simulink model "KUKA_LUNGU"  (R2016b)
settings: Solver=VariableStepAuto  StartTime=0  StopTime=inf  RelTol=1e-3
undefined symbols (not defined in the file or in its folder): KR16, KR16L1, KR16L2, KR16L3, KR16L4, KR16L5, KR16L6, KR16底座, KR16电主轴, KUKA, RootGround, RootPart
libraries: mblibv1 x42, simulink x7
settings Model: Creator=16591  LastModifiedBy=16591
settings SimMechanicsCC: VisOnUpdateDiagram=on  VisDuringSimulation=on

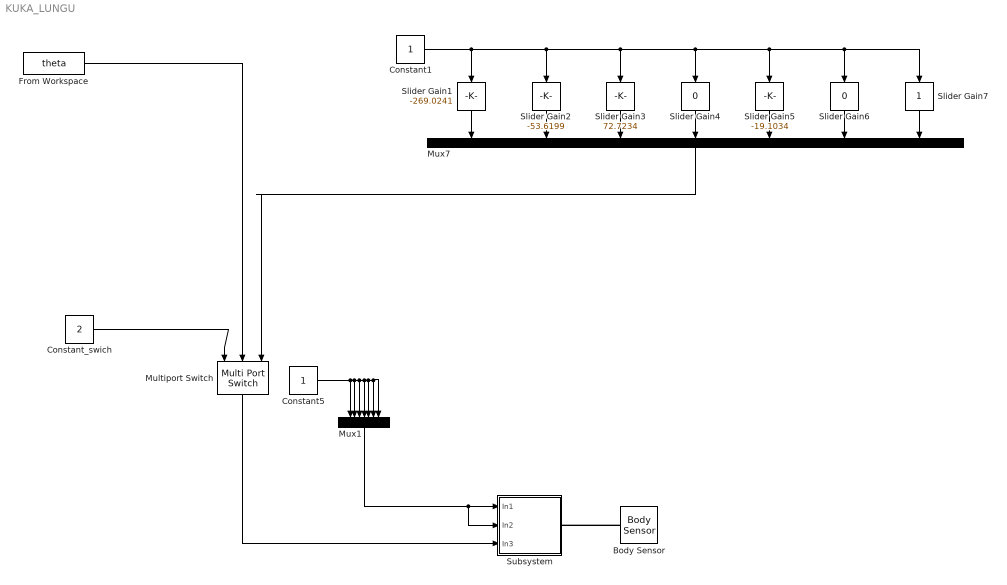
== system KUKA_LUNGU ==
  Body Sensor : mblibv1/Sensors &  Actuators/Body Sensor  UpdateFromCAD=off  PhysicalDomain=Mechanical  PortType=blob  Muxed=on  Pose=off  Angle=on  AngleUnits=deg  ArcVelocity=off  ArcVelocityUnits=deg/s  ArcAcceleration=off  ArcAccelerationUnits=deg/s^2  CoordPosition=on  CoordPositionUnits=m  Velocity=off  VelocityUnits=m/s  Acceleration=off  AccelerationUnits=m/s^2  Quaternion=on  QuaternionDT=off  QuaternionDDT=off  QuaternionUnits=off  OutputVector=[1]  ActiveIO=on  Width=3  DialogClass=MechanicalSensorBlock  ReferenceFrame=Absolute (World)
  Constant1 : Constant
  Constant5 : Constant
  Constant_swich : Constant  Value=2
  From Workspace : FromWorkspace  VariableName=theta  SampleTime=0.1
  Multiport Switch : MultiPortSwitch  Inputs=2
  Mux1 : Mux  Inputs=7
  Mux7 : Mux  Inputs=7
  Slider Gain1 : simulink/Math Operations/Slider Gain  low=-185  gain=-269.0241  high=185
  Slider Gain2 : simulink/Math Operations/Slider Gain  low=-155  gain=-53.6199  high=35
  Slider Gain3 : simulink/Math Operations/Slider Gain  low=-130  gain=72.7234  high=154
  Slider Gain4 : simulink/Math Operations/Slider Gain  low=-350  gain=0  high=350
  Slider Gain5 : simulink/Math Operations/Slider Gain  low=-130  gain=-19.1034  high=130
  Slider Gain6 : simulink/Math Operations/Slider Gain  low=-350  gain=0  high=350
  Slider Gain7 : simulink/Math Operations/Slider Gain  low=0  gain=1  high=2
  Subsystem : Subsystem
  wires:
  Multiport Switch/1 -> Subsystem/3(In3)
  Slider Gain1/1 -> Mux7/1
  Constant1/1 -> Slider Gain7/1, Slider Gain6/1, Slider Gain5/1, Slider Gain4/1, Slider Gain3/1, Slider Gain2/1, Slider Gain1/1
  Slider Gain2/1 -> Mux7/2
  Slider Gain3/1 -> Mux7/3
  Slider Gain4/1 -> Mux7/4
  Slider Gain5/1 -> Mux7/5
  Slider Gain6/1 -> Mux7/6
  Slider Gain7/1 -> Mux7/7
  Mux7/1 -> Multiport Switch/3
  Constant_swich/1 -> Multiport Switch/1
  Constant5/1 -> Mux1/1, Mux1/7, Mux1/6, Mux1/5, Mux1/4, Mux1/3, Mux1/2
  Mux1/1 -> Subsystem/2(In2), Subsystem/1(In1)
  From Workspace/1 -> Multiport Switch/2
  connections:
  Body Sensor/LConn1 -- Subsystem/RConn1

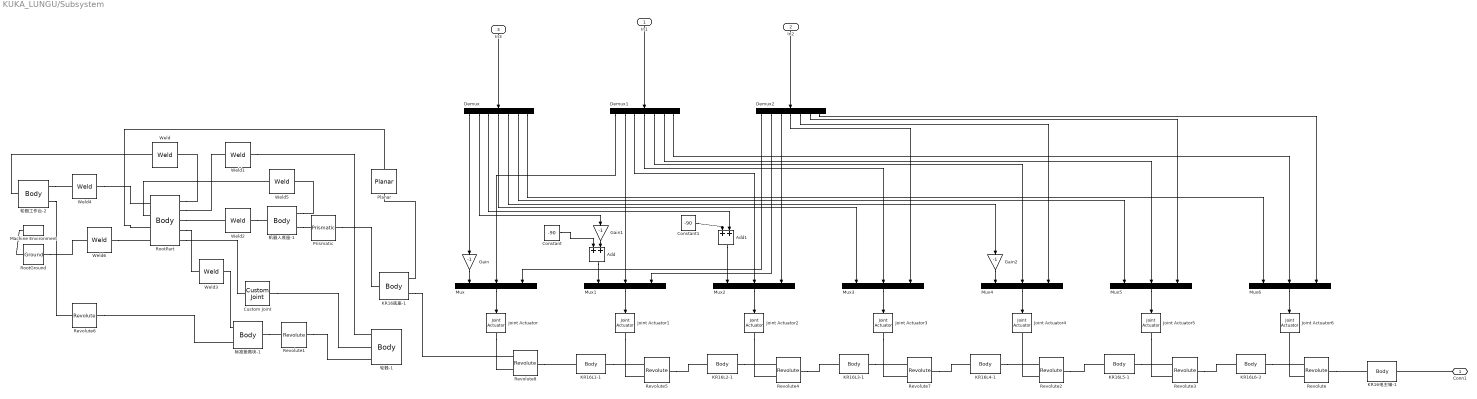
== system KUKA_LUNGU/Subsystem ==
  In1 : Inport
  In2 : Inport  Port=2
  In3 : Inport  Port=3
  Add : Sum
  Add1 : Sum
  Constant : Constant  Value=-90
  Constant1 : Constant  Value=-90
  Custom Joint : mblibv1/Joints/Custom Joint  LConnTagsString=__newl0  RConnTagsString=__newr0  UpdateFromCAD=on  PMImportedID=:-:KUKA-KR16-汽车轮毂/RootPart  NumSAPorts=0  CutJoint=off  MarkAsCut=off  Primitives=prismatic  PrimitiveProps=P1$WORLD$[1,0,0]$prismatic#P2$WORLD$[0,1,0]$prismatic#P3$WORLD$[0,0,1]$prismatic#R1$WORLD$[1,0,0]$revolute  DialogClass=JointBlock  R1Axis=[1,0,0]  R2Axis=[]  R3Axis=[]  P1Axis=[1,0,0]  P2Axis=[0,1,0]  P3Axis=[0,0,1]  SAxis=[]
  Demux : Demux  Outputs=7
  Demux1 : Demux  Outputs=7
  Demux2 : Demux  Outputs=7
  Gain : Gain  Gain=-1
  Gain1 : Gain  Gain=-1
  Gain2 : Gain  Gain=-1
  Joint Actuator{,1..6} (7 alike) : mblibv1/Sensors &  Actuators/Joint Actuator  UpdateFromCAD=off  PhysicalDomain=Mechanical  PortType=blob  ActuationStyle=Motion  AngleUnits=deg  ArcVelocityUnits=deg/s  ArcAccelerationUnits=deg/s^2  CoordPositionUnits=m  VelocityUnits=m/s  AccelerationUnits=m/s^2  ForceUnits=N  TorqueUnits=N*m  ActiveIO=on  Width=3  DialogClass=MechanicalActuatorBlock  Primitive=R1  ReferenceFrame=Absolute (World)
  KR16L1-1 : mblibv1/Bodies/Body  LConnTagsString=CS3  RConnTagsString=CS2  UpdateFromCAD=on  PMImportedID=KR16L1-1  DialogClass=MechanicalBodyBlock  Mass=25.8177  MassUnits=kg  InertiaUnits=kg*m^2  Inertia=[0.576803,-0.0576744,-0.301475;-0.0576744,0.906894,-0.0524576;-0.301475,-0.0524576,0.799958]  Shape=Cylinder  ShapeDims=[1 1]  ShapeUnits=m  ShapeUse=false  Density=1  DensityUnits=kg/m^3  DensityUse=false  GraphicsMode=GFXFILE  GraphicsFileName=KUKA-KR16-汽车轮毂 - KR16L1-1.STL  BodyColorSelMode=COLORPALETTE  BodyColor=[0.960784;0.419608;0.141176]  AttachedToCS=CS1  CG=Right$CG$[0.119444 1.06418 -0.0189084]$WORLD$WORLD$m$[1 0 0;0 0 1;0 -1 0]$3x3 Transform$rad$WORLD$false$KR16L1-1::CG(AUTOGEN)  WorkingFrames=Right$CS1$[0 0.5 0]$WORLD$WORLD$m$[1 0 0;0 0 1;0 -1 0]$3x3 Transform$rad$WORLD$false$KR16L1-1::CS1(AUTOGEN)#Right$CS2$[0.26 1.175 0.067]$WORLD$WORLD$m$[1 0 0;0 1 0;0 0 1]$3x3 Transform$rad$WORLD$true$KR16L1-1:-:KR16L2-1::KR16L1-1(AUTOGEN)#Left$CS3$[0 0.5474 0]$WORLD$WORLD$m$[1 0 0;0 1 0;0 0 1]$3x3 Transform$rad$WORLD$true$KR16L1-1:-:KR16底座-1::KR16L1-1(AUTOGEN)  CGPos=[0.119444 1.06418 -0.0189084]  CGRot=[1 0 0;0 0 1;0 -1 0]  CS0Pos=[]  CS0Rot=[]  CS1Pos=[0 0.5 0]  CS1Rot=[1 0 0;0 0 1;0 -1 0]  CS2Pos=[0.26 1.175 0.067]  CS2Rot=[1 0 0;0 1 0;0 0 1]  CS3Pos=[0 0.5474 0]  CS3Rot=[1 0 0;0 1 0;0 0 1]  CS4Pos=[]  CS4Rot=[]  CS5Pos=[]  CS5Rot=[]  CS6Pos=[]  CS6Rot=[]  CS7Pos=[]  CS7Rot=[]  CS8Pos=[]  CS8Rot=[]  CS9Pos=[]  CS9Rot=[]  CS10Pos=[]  CS10Rot=[]  CS11Pos=[]  CS11Rot=[]  CS12Pos=[]  CS12Rot=[]  CS13Pos=[]  CS13Rot=[]  CS14Pos=[]  CS14Rot=[]  CS15Pos=[]  CS15Rot=[]  CS16Pos=[]  CS16Rot=[]  CS17Pos=[]  CS17Rot=[]  CS18Pos=[]  CS18Rot=[]  CS19Pos=[]  CS19Rot=[]  CS20Pos=[]  CS20Rot=[]
  KR16L2-1 : mblibv1/Bodies/Body  LConnTagsString=CS3  RConnTagsString=CS2  UpdateFromCAD=on  PMImportedID=KR16L2-1  DialogClass=MechanicalBodyBlock  Mass=13.4955  MassUnits=kg  InertiaUnits=kg*m^2  Inertia=[0.593067,-0.000241705,-0.000338834;-0.000241705,0.591348,0.0261399;-0.000338834,0.0261399,0.0591147]  Shape=Cylinder  ShapeDims=[1 1]  ShapeUnits=m  ShapeUse=false  Density=1  DensityUnits=kg/m^3  DensityUse=false  GraphicsMode=GFXFILE  GraphicsFileName=KUKA-KR16-汽车轮毂 - KR16L2-1.STL  BodyColorSelMode=COLORPALETTE  BodyColor=[0.960784;0.419608;0.141176]  AttachedToCS=CS1  CG=Right$CG$[0.260237 1.49663 0.180665]$WORLD$WORLD$m$[1 0 -5.63789e-11;5.63789e-11 0 1;0 -1 0]$3x3 Transform$rad$WORLD$false$KR16L2-1::CG(AUTOGEN)  WorkingFrames=Right$CS1$[3.8056e-11 0.5 0]$WORLD$WORLD$m$[1 0 -5.63789e-11;5.63789e-11 0 1;0 -1 0]$3x3 Transform$rad$WORLD$false$KR16L2-1::CS1(AUTOGEN)#Right$CS2$[0.26 1.855 0.107]$WORLD$WORLD$m$[1 0 0;0 1 0;0 0 1]$3x3 Transform$rad$WORLD$true$KR16L2-1:-:KR16L3-1::KR16L2-1(AUTOGEN)#Left$CS3$[0.26 1.175 0.067]$WORLD$WORLD$m$[1 0 0;0 1 0;0 0 1]$3x3 Transform$rad$WORLD$true$KR16L1-1:-:KR16L2-1::KR16L2-1(AUTOGEN)  CGPos=[0.260237 1.49663 0.180665]  CGRot=[1 0 -5.63789e-11;5.63789e-11 0 1;0 -1 0]  CS0Pos=[]  CS0Rot=[]  CS1Pos=[3.8056e-11 0.5 0]  CS1Rot=[1 0 -5.63789e-11;5.63789e-11 0 1;0 -1 0]  CS2Pos=[0.26 1.855 0.107]  CS2Rot=[1 0 0;0 1 0;0 0 1]  CS3Pos=[0.26 1.175 0.067]  CS3Rot=[1 0 0;0 1 0;0 0 1]  CS4Pos=[]  CS4Rot=[]  CS5Pos=[]  CS5Rot=[]  CS6Pos=[]  CS6Rot=[]  CS7Pos=[]  CS7Rot=[]  CS8Pos=[]  CS8Rot=[]  CS9Pos=[]  CS9Rot=[]  CS10Pos=[]  CS10Rot=[]  CS11Pos=[]  CS11Rot=[]  CS12Pos=[]  CS12Rot=[]  CS13Pos=[]  CS13Rot=[]  CS14Pos=[]  CS14Rot=[]  CS15Pos=[]  CS15Rot=[]  CS16Pos=[]  CS16Rot=[]  CS17Pos=[]  CS17Rot=[]  CS18Pos=[]  CS18Rot=[]  CS19Pos=[]  CS19Rot=[]  CS20Pos=[]  CS20Rot=[]
  KR16L3-1 : mblibv1/Bodies/Body  LConnTagsString=CS2  RConnTagsString=CS3  UpdateFromCAD=on  PMImportedID=KR16L3-1  DialogClass=MechanicalBodyBlock  Mass=16.2699  MassUnits=kg  InertiaUnits=kg*m^2  Inertia=[0.125403,0.00230248,0.000189371;0.00230248,0.543915,-0.00277001;0.000189371,-0.00277001,0.558145]  Shape=Cylinder  ShapeDims=[1 1]  ShapeUnits=m  ShapeUse=false  Density=1  DensityUnits=kg/m^3  DensityUse=false  GraphicsMode=GFXFILE  GraphicsFileName=KUKA-KR16-汽车轮毂 - KR16L3-1.STL  BodyColorSelMode=COLORPALETTE  BodyColor=[0.960784;0.419608;0.141176]  AttachedToCS=CS1  CG=Right$CG$[0.262138 1.83547 -0.00994259]$WORLD$WORLD$m$[1 0 -6.72099e-11;6.72099e-11 0 1;0 -1 0]$3x3 Transform$rad$WORLD$false$KR16L3-1::CG(AUTOGEN)  WorkingFrames=Right$CS1$[5.2732e-11 0.5 0]$WORLD$WORLD$m$[1 0 -6.72099e-11;6.72099e-11 0 1;0 -1 0]$3x3 Transform$rad$WORLD$false$KR16L3-1::CS1(AUTOGEN)#Left$CS2$[0.26 1.855 0.107]$WORLD$WORLD$m$[1 0 0;0 1 0;0 0 1]$3x3 Transform$rad$WORLD$true$KR16L2-1:-:KR16L3-1::KR16L3-1(AUTOGEN)#Right$CS3$[0.111 1.82 0]$WORLD$WORLD$m$[1 0 0;0 1 0;0 0 1]$3x3 Transform$rad$WORLD$true$KR16L3-1:-:KR16L4-1::KR16L3-1(AUTOGEN)  CGPos=[0.262138 1.83547 -0.00994259]  CGRot=[1 0 -6.72099e-11;6.72099e-11 0 1;0 -1 0]  CS0Pos=[]  CS0Rot=[]  CS1Pos=[5.2732e-11 0.5 0]  CS1Rot=[1 0 -6.72099e-11;6.72099e-11 0 1;0 -1 0]  CS2Pos=[0.26 1.855 0.107]  CS2Rot=[1 0 0;0 1 0;0 0 1]  CS3Pos=[0.111 1.82 0]  CS3Rot=[1 0 0;0 1 0;0 0 1]  CS4Pos=[]  CS4Rot=[]  CS5Pos=[]  CS5Rot=[]  CS6Pos=[]  CS6Rot=[]  CS7Pos=[]  CS7Rot=[]  CS8Pos=[]  CS8Rot=[]  CS9Pos=[]  CS9Rot=[]  CS10Pos=[]  CS10Rot=[]  CS11Pos=[]  CS11Rot=[]  CS12Pos=[]  CS12Rot=[]  CS13Pos=[]  CS13Rot=[]  CS14Pos=[]  CS14Rot=[]  CS15Pos=[]  CS15Rot=[]  CS16Pos=[]  CS16Rot=[]  CS17Pos=[]  CS17Rot=[]  CS18Pos=[]  CS18Rot=[]  CS19Pos=[]  CS19Rot=[]  CS20Pos=[]  CS20Rot=[]
  KR16L4-1 : mblibv1/Bodies/Body  LConnTagsString=CS3  RConnTagsString=CS2  UpdateFromCAD=on  PMImportedID=KR16L4-1  DialogClass=MechanicalBodyBlock  Mass=3.83148  MassUnits=kg  InertiaUnits=kg*m^2  Inertia=[0.00881654,-0.00289828,3.03725e-06;-0.00289828,0.0376269,-2.2375e-05;3.03725e-06,-2.2375e-05,0.0382811]  Shape=Cylinder  ShapeDims=[1 1]  ShapeUnits=m  ShapeUse=false  Density=1  DensityUnits=kg/m^3  DensityUse=false  GraphicsMode=GFXFILE  GraphicsFileName=KUKA-KR16-汽车轮毂 - KR16L4-1.STL  BodyColorSelMode=COLORPALETTE  BodyColor=[0.960784;0.419608;0.141176]  AttachedToCS=CS1  CG=Right$CG$[0.794534 1.81999 -0.00555632]$WORLD$WORLD$m$[1 0 -6.72102e-11;6.72101e-11 -5.18527e-12 1;0 -1 -5.18528e-12]$3x3 Transform$rad$WORLD$false$KR16L4-1::CG(AUTOGEN)  WorkingFrames=Right$CS1$[5.27326e-11 0.5 7.41978e-12]$WORLD$WORLD$m$[1 0 -6.72102e-11;6.72101e-11 -5.18527e-12 1;0 -1 -5.18528e-12]$3x3 Transform$rad$WORLD$false$KR16L4-1::CS1(AUTOGEN)#Right$CS2$[0.93 1.82 0.0335]$WORLD$WORLD$m$[1 0 0;0 1 0;0 0 1]$3x3 Transform$rad$WORLD$true$KR16L4-1:-:KR16L5-1::KR16L4-1(AUTOGEN)#Left$CS3$[0.111 1.82 0]$WORLD$WORLD$m$[1 0 0;0 1 0;0 0 1]$3x3 Transform$rad$WORLD$true$KR16L3-1:-:KR16L4-1::KR16L4-1(AUTOGEN)  CGPos=[0.794534 1.81999 -0.00555632]  CGRot=[1 0 -6.72102e-11;6.72101e-11 -5.18527e-12 1;0 -1 -5.18528e-12]  CS0Pos=[]  CS0Rot=[]  CS1Pos=[5.27326e-11 0.5 7.41978e-12]  CS1Rot=[1 0 -6.72102e-11;6.72101e-11 -5.18527e-12 1;0 -1 -5.18528e-12]  CS2Pos=[0.93 1.82 0.0335]  CS2Rot=[1 0 0;0 1 0;0 0 1]  CS3Pos=[0.111 1.82 0]  CS3Rot=[1 0 0;0 1 0;0 0 1]  CS4Pos=[]  CS4Rot=[]  CS5Pos=[]  CS5Rot=[]  CS6Pos=[]  CS6Rot=[]  CS7Pos=[]  CS7Rot=[]  CS8Pos=[]  CS8Rot=[]  CS9Pos=[]  CS9Rot=[]  CS10Pos=[]  CS10Rot=[]  CS11Pos=[]  CS11Rot=[]  CS12Pos=[]  CS12Rot=[]  CS13Pos=[]  CS13Rot=[]  CS14Pos=[]  CS14Rot=[]  CS15Pos=[]  CS15Rot=[]  CS16Pos=[]  CS16Rot=[]  CS17Pos=[]  CS17Rot=[]  CS18Pos=[]  CS18Rot=[]  CS19Pos=[]  CS19Rot=[]  CS20Pos=[]  CS20Rot=[]
  KR16L5-1 : mblibv1/Bodies/Body  LConnTagsString=CS2  RConnTagsString=CS3  UpdateFromCAD=on  PMImportedID=KR16L5-1  DialogClass=MechanicalBodyBlock  Mass=1.85731  MassUnits=kg  InertiaUnits=kg*m^2  Inertia=[0.008719,0.000329435,2.41862e-07;0.000329435,0.00689293,-1.21594e-06;2.41862e-07,-1.21594e-06,0.012927]  Shape=Cylinder  ShapeDims=[1 1]  ShapeUnits=m  ShapeUse=false  Density=1  DensityUnits=kg/m^3  DensityUse=false  GraphicsMode=GFXFILE  GraphicsFileName=KUKA-KR16-汽车轮毂 - KR16L5-1.STL  BodyColorSelMode=COLORPALETTE  BodyColor=[0.960784;0.419608;0.141176]  AttachedToCS=CS1  CG=Right$CG$[0.930049 1.7697 0.0071318]$WORLD$WORLD$m$[4.40623e-11 1.89374e-10 1;-1 -5.18503e-12 4.40623e-11;5.18503e-12 -1 1.89374e-10]$3x3 Transform$rad$WORLD$false$KR16L5-1::CG(AUTOGEN)  WorkingFrames=Right$CS1$[-0.39 2.75 -2.54769e-10]$WORLD$WORLD$m$[4.40623e-11 1.89374e-10 1;-1 -5.18503e-12 4.40623e-11;5.18503e-12 -1 1.89374e-10]$3x3 Transform$rad$WORLD$false$KR16L5-1::CS1(AUTOGEN)#Left$CS2$[0.93 1.82 0.0335]$WORLD$WORLD$m$[1 0 0;0 1 0;0 0 1]$3x3 Transform$rad$WORLD$true$KR16L4-1:-:KR16L5-1::KR16L5-1(AUTOGEN)#Right$CS3$[0.93 1.662 7.32896e-11]$WORLD$WORLD$m$[1 0 0;0 1 0;0 0 1]$3x3 Transform$rad$WORLD$true$KR16L5-1:-:KR16L6-3::KR16L5-1(AUTOGEN)  CGPos=[0.930049 1.7697 0.0071318]  CGRot=[4.40623e-11 1.89374e-10 1;-1 -5.18503e-12 4.40623e-11;5.18503e-12 -1 1.89374e-10]  CS0Pos=[]  CS0Rot=[]  CS1Pos=[-0.39 2.75 -2.54769e-10]  CS1Rot=[4.40623e-11 1.89374e-10 1;-1 -5.18503e-12 4.40623e-11;5.18503e-12 -1 1.89374e-10]  CS2Pos=[0.93 1.82 0.0335]  CS2Rot=[1 0 0;0 1 0;0 0 1]  CS3Pos=[0.93 1.662 7.32896e-11]  CS3Rot=[1 0 0;0 1 0;0 0 1]  CS4Pos=[]  CS4Rot=[]  CS5Pos=[]  CS5Rot=[]  CS6Pos=[]  CS6Rot=[]  CS7Pos=[]  CS7Rot=[]  CS8Pos=[]  CS8Rot=[]  CS9Pos=[]  CS9Rot=[]  CS10Pos=[]  CS10Rot=[]  CS11Pos=[]  CS11Rot=[]  CS12Pos=[]  CS12Rot=[]  CS13Pos=[]  CS13Rot=[]  CS14Pos=[]  CS14Rot=[]  CS15Pos=[]  CS15Rot=[]  CS16Pos=[]  CS16Rot=[]  CS17Pos=[]  CS17Rot=[]  CS18Pos=[]  CS18Rot=[]  CS19Pos=[]  CS19Rot=[]  CS20Pos=[]  CS20Rot=[]
  KR16L6-3 : mblibv1/Bodies/Body  LConnTagsString=CS3  RConnTagsString=CS2  UpdateFromCAD=on  PMImportedID=KR16L6-3  DialogClass=MechanicalBodyBlock  Mass=1.24036  MassUnits=kg  InertiaUnits=kg*m^2  Inertia=[0.00519585,0,0;0,0.00167069,0;0,0,0.00515745]  Shape=Cylinder  ShapeDims=[1 1]  ShapeUnits=m  ShapeUse=false  Density=1  DensityUnits=kg/m^3  DensityUse=false  GraphicsMode=GFXFILE  GraphicsFileName=KUKA-KR16-汽车轮毂 - KR16L6-3.STL  BodyColorSelMode=COLORPALETTE  BodyColor=[0.529412;0.54902;0.54902]  AttachedToCS=CS1  CG=Right$CG$[0.93 1.57551 7.3738e-11]$WORLD$WORLD$m$[0 -4.40624e-11 -1;5.1849e-12 1 -4.40623e-11;1 -5.18491e-12 0]$3x3 Transform$rad$WORLD$false$KR16L6-3::CG(AUTOGEN)  WorkingFrames=Right$CS1$[0.93 1.462 7.43266e-11]$WORLD$WORLD$m$[0 -4.40624e-11 -1;5.1849e-12 1 -4.40623e-11;1 -5.18491e-12 0]$3x3 Transform$rad$WORLD$false$KR16L6-3::CS1(AUTOGEN)#Right$CS2$[0.93 1.618 7.35177e-11]$WORLD$WORLD$m$[1 0 0;0 1 0;0 0 1]$3x3 Transform$rad$WORLD$true$KR16L6-3:-:KR16电主轴-1::KR16L6-3(AUTOGEN)#Left$CS3$[0.93 1.662 7.32896e-11]$WORLD$WORLD$m$[1 0 0;0 1 0;0 0 1]$3x3 Transform$rad$WORLD$true$KR16L5-1:-:KR16L6-3::KR16L6-3(AUTOGEN)  CGPos=[0.93 1.57551 7.3738e-11]  CGRot=[0 -4.40624e-11 -1;5.1849e-12 1 -4.40623e-11;1 -5.18491e-12 0]  CS0Pos=[]  CS0Rot=[]  CS1Pos=[0.93 1.462 7.43266e-11]  CS1Rot=[0 -4.40624e-11 -1;5.1849e-12 1 -4.40623e-11;1 -5.18491e-12 0]  CS2Pos=[0.93 1.618 7.35177e-11]  CS2Rot=[1 0 0;0 1 0;0 0 1]  CS3Pos=[0.93 1.662 7.32896e-11]  CS3Rot=[1 0 0;0 1 0;0 0 1]  CS4Pos=[]  CS4Rot=[]  CS5Pos=[]  CS5Rot=[]  CS6Pos=[]  CS6Rot=[]  CS7Pos=[]  CS7Rot=[]  CS8Pos=[]  CS8Rot=[]  CS9Pos=[]  CS9Rot=[]  CS10Pos=[]  CS10Rot=[]  CS11Pos=[]  CS11Rot=[]  CS12Pos=[]  CS12Rot=[]  CS13Pos=[]  CS13Rot=[]  CS14Pos=[]  CS14Rot=[]  CS15Pos=[]  CS15Rot=[]  CS16Pos=[]  CS16Rot=[]  CS17Pos=[]  CS17Rot=[]  CS18Pos=[]  CS18Rot=[]  CS19Pos=[]  CS19Rot=[]  CS20Pos=[]  CS20Rot=[]
  KR16底座-1 : mblibv1/Bodies/Body  LConnTagsString=CS3  RConnTagsString=CS2|CS4  UpdateFromCAD=on  PMImportedID=KR16底座-1  DialogClass=MechanicalBodyBlock  Mass=70.1358  MassUnits=kg  InertiaUnits=kg*m^2  Inertia=[1.74612,0.032286,-0.0123849;0.032286,2.12719,-0.000120145;-0.0123849,-0.000120145,2.2593]  Shape=Cylinder  ShapeDims=[1 1]  ShapeUnits=m  ShapeUse=false  Density=1  DensityUnits=kg/m^3  DensityUse=false  GraphicsMode=GFXFILE  GraphicsFileName=KUKA-KR16-汽车轮毂 - KR16底座-1.STL  BodyColorSelMode=COLORPALETTE  BodyColor=[0.14902;0.14902;0.14902]  AttachedToCS=CS1  CG=Right$CG$[-0.0392869 0.697192 -0.00150494]$WORLD$WORLD$m$[1 0 0;0 0 1;0 -1 0]$3x3 Transform$rad$WORLD$false$KR16底座-1::CG(AUTOGEN)  WorkingFrames=Right$CS1$[0 0.5 0]$WORLD$WORLD$m$[1 0 0;0 0 1;0 -1 0]$3x3 Transform$rad$WORLD$false$KR16底座-1::CS1(AUTOGEN)#Right$CS2$[0 0.5 0]$WORLD$WORLD$m$[1 0 0;0 1 0;0 0 1]$3x3 Transform$rad$WORLD$true$:-:KUKA-KR16-汽车轮毂/RootPart::KR16底座-1(AUTOGEN)#Left$CS3$[0 0.5 0]$WORLD$WORLD$m$[1 0 0;0 1 0;0 0 1]$3x3 Transform$rad$WORLD$true$KR16底座-1:-:机器人底座-1::KR16底座-1(AUTOGEN)#Right$CS4$[0 0.5474 0]$WORLD$WORLD$m$[1 0 0;0 1 0;0 0 1]$3x3 Transform$rad$WORLD$true$KR16L1-1:-:KR16底座-1::KR16底座-1(AUTOGEN)  CGPos=[-0.0392869 0.697192 -0.00150494]  CGRot=[1 0 0;0 0 1;0 -1 0]  CS0Pos=[]  CS0Rot=[]  CS1Pos=[0 0.5 0]  CS1Rot=[1 0 0;0 0 1;0 -1 0]  CS2Pos=[0 0.5 0]  CS2Rot=[1 0 0;0 1 0;0 0 1]  CS3Pos=[0 0.5 0]  CS3Rot=[1 0 0;0 1 0;0 0 1]  CS4Pos=[0 0.5474 0]  CS4Rot=[1 0 0;0 1 0;0 0 1]  CS5Pos=[]  CS5Rot=[]  CS6Pos=[]  CS6Rot=[]  CS7Pos=[]  CS7Rot=[]  CS8Pos=[]  CS8Rot=[]  CS9Pos=[]  CS9Rot=[]  CS10Pos=[]  CS10Rot=[]  CS11Pos=[]  CS11Rot=[]  CS12Pos=[]  CS12Rot=[]  CS13Pos=[]  CS13Rot=[]  CS14Pos=[]  CS14Rot=[]  CS15Pos=[]  CS15Rot=[]  CS16Pos=[]  CS16Rot=[]  CS17Pos=[]  CS17Rot=[]  CS18Pos=[]  CS18Rot=[]  CS19Pos=[]  CS19Rot=[]  CS20Pos=[]  CS20Rot=[]
  KR16电主轴-1 : mblibv1/Bodies/Body  LConnTagsString=CS2  RConnTagsString=CS3  UpdateFromCAD=on  PMImportedID=KR16电主轴-1  DialogClass=MechanicalBodyBlock  Mass=0.0101259  MassUnits=kg  InertiaUnits=kg*m^2  Inertia=[2.07229e-06,0,0;0,4.76675e-07,0;0,0,2.07229e-06]  Shape=Cylinder  ShapeDims=[1 1]  ShapeUnits=m  ShapeUse=false  Density=1  DensityUnits=kg/m^3  DensityUse=false  GraphicsMode=GFXFILE  GraphicsFileName=KUKA-KR16-汽车轮毂 - KR16电主轴-1.STL  BodyColorSelMode=COLORPALETTE  BodyColor=[1;0;0]  AttachedToCS=CS1  CG=Right$CG$[0.93 1.44419 7.44189e-11]$WORLD$WORLD$m$[-0.760403 -4.40624e-11 -0.649452;-3.01378e-11 1 -3.2559e-11;0.649452 -5.18491e-12 -0.760403]$3x3 Transform$rad$WORLD$false$KR16电主轴-1::CG(AUTOGEN)  WorkingFrames=Right$CS3$[0.93 1.44419 7.44189e-11]$WORLD$WORLD$m$[-0.760403 -4.40624e-11 -0.649452;-3.01378e-11 1 -3.2559e-11;0.649452 -5.18491e-12 -0.760403]$3x3 Transform$rad$WORLD$true$none#Right$CS1$[0.93 1.402 7.46377e-11]$WORLD$WORLD$m$[-0.760403 -4.40624e-11 -0.649452;-3.01378e-11 1 -3.2559e-11;0.649452 -5.18491e-12 -0.760403]$3x3 Transform$rad$WORLD$false$KR16电主轴-1::CS1(AUTOGEN)#Left$CS2$[0.93 1.618 7.35177e-11]$WORLD$WORLD$m$[1 0 0;0 1 0;0 0 1]$3x3 Transform$rad$WORLD$true$KR16L6-3:-:KR16电主轴-1::KR16电主轴-1(AUTOGEN)  CGPos=[0.93 1.44419 7.44189e-11]  CGRot=[-0.760403 -4.40624e-11 -0.649452;-3.01378e-11 1 -3.2559e-11;0.649452 -5.18491e-12 -0.760403]  CS0Pos=[]  CS0Rot=[]  CS1Pos=[0.93 1.402 7.46377e-11]  CS1Rot=[-0.760403 -4.40624e-11 -0.649452;-3.01378e-11 1 -3.2559e-11;0.649452 -5.18491e-12 -0.760403]  CS2Pos=[0.93 1.618 7.35177e-11]  CS2Rot=[1 0 0;0 1 0;0 0 1]  CS3Pos=[0.93 1.44419 7.44189e-11]  CS3Rot=[-0.760403 -4.40624e-11 -0.649452;-3.01378e-11 1 -3.2559e-11;0.649452 -5.18491e-12 -0.760403]  CS4Pos=[]  CS4Rot=[]  CS5Pos=[]  CS5Rot=[]  CS6Pos=[]  CS6Rot=[]  CS7Pos=[]  CS7Rot=[]  CS8Pos=[]  CS8Rot=[]  CS9Pos=[]  CS9Rot=[]  CS10Pos=[]  CS10Rot=[]  CS11Pos=[]  CS11Rot=[]  CS12Pos=[]  CS12Rot=[]  CS13Pos=[]  CS13Rot=[]  CS14Pos=[]  CS14Rot=[]  CS15Pos=[]  CS15Rot=[]  CS16Pos=[]  CS16Rot=[]  CS17Pos=[]  CS17Rot=[]  CS18Pos=[]  CS18Rot=[]  CS19Pos=[]  CS19Rot=[]  CS20Pos=[]  CS20Rot=[]
  Machine Environment : mblibv1/Bodies/Machine Environment  PortType=env  PhysicalDomain=Mechanical  DialogTemplateClass=MECH.MachineEnvironment  SyncWhenCopied=off  Gravity=[0 -9.81 0]  GravityUnits=m/s^2  GravityAsSignal=off  Dimensionality=Auto-detect  AnalysisType=Forward dynamics  LinearAssemblyTolerance=1e-3  LinearAssemblyToleranceUnits=m  AngularAssemblyTolerance=1e-3  AngularAssemblyToleranceUnits=rad  ConstraintSolverType=Stabilizing  ConstraintRelTolerance=1e-4  ConstraintAbsTolerance=1e-4  UseRobustSingularityHandling=off  RedundancyAnalysisToleranceType=Automatically select tolerance  RedundancyAnalysisTolerance=1e-14  StatePerturbationType=Fixed  PerturbationSize=1e-5  VisualizeMachine=on  BodyVisualizationType=Use model default body geometries  BodyColorSelMode=Use model default  DefaultBodyColor=[1 0 0]
  Mux{,1..6} (7 alike) : Mux  Inputs=3
  Planar : mblibv1/Joints/Planar  LConnTagsString=__newl0  RConnTagsString=__newr0  UpdateFromCAD=on  PMImportedID=:-:KUKA-KR16-汽车轮毂/RootPart  NumSAPorts=0  CutJoint=off  MarkAsCut=off  Primitives=prismatic_prismatic  PrimitiveProps=P1$WORLD$[-1,0,0]$prismatic#P2$WORLD$[0,-1,0]$prismatic#R1$WORLD$[0,0,-1]$revolute  DialogClass=JointBlock  P1Axis=[-1,0,0]  P2Axis=[0,-1,0]  R1Axis=[0,0,-1]
  Prismatic : mblibv1/Joints/Prismatic  LConnTagsString=__newl0  RConnTagsString=__newr0  UpdateFromCAD=on  PMImportedID=KR16底座-1:-:机器人底座-1  NumSAPorts=0  CutJoint=off  MarkAsCut=off  Primitives=prismatic  PrimitiveProps=P1$WORLD$[0,0,1]$prismatic  DialogClass=JointBlock  P1Axis=[0,0,1]
  Revolute : mblibv1/Joints/Revolute  LConnTagsString=__newl0|SA1  RConnTagsString=__newr0  UpdateFromCAD=on  PMImportedID=KR16L6-3:-:KR16电主轴-1  NumSAPorts=1  CutJoint=off  MarkAsCut=off  Primitives=prismatic  PrimitiveProps=R1$World$[4.40624e-11,-1,5.18492e-12]$revolute  DialogClass=JointBlock  R1Axis=[4.40624e-11,-1,5.18492e-12]
  Revolute1 : mblibv1/Joints/Revolute  LConnTagsString=__newl0  RConnTagsString=__newr0  UpdateFromCAD=on  PMImportedID=标准垫高块-1:-:轮毂-1  NumSAPorts=0  CutJoint=off  MarkAsCut=off  Primitives=prismatic  PrimitiveProps=R1$WORLD$[0,1,0]$revolute  DialogClass=JointBlock  R1Axis=[0,1,0]
  Revolute2 : mblibv1/Joints/Revolute  LConnTagsString=__newl0|SA1  RConnTagsString=__newr0  UpdateFromCAD=on  PMImportedID=KR16L4-1:-:KR16L5-1  NumSAPorts=1  CutJoint=off  MarkAsCut=off  Primitives=prismatic  PrimitiveProps=R1$World$[-1.89374e-10,5.18525e-12,1]$revolute  DialogClass=JointBlock  R1Axis=[-1.89374e-10,5.18525e-12,1]
  Revolute3 : mblibv1/Joints/Revolute  LConnTagsString=__newl0|SA1  RConnTagsString=__newr0  UpdateFromCAD=on  PMImportedID=KR16L5-1:-:KR16L6-3  NumSAPorts=1  CutJoint=off  MarkAsCut=off  Primitives=prismatic  PrimitiveProps=R1$World$[-4.40623e-11,1,-5.18503e-12]$revolute  DialogClass=JointBlock  R1Axis=[-4.40623e-11,1,-5.18503e-12]
  Revolute4 : mblibv1/Joints/Revolute  LConnTagsString=__newl0|SA1  RConnTagsString=__newr0  UpdateFromCAD=on  PMImportedID=KR16L2-1:-:KR16L3-1  NumSAPorts=1  CutJoint=off  MarkAsCut=off  Primitives=prismatic  PrimitiveProps=R1$World$[0,0,-1]$revolute  DialogClass=JointBlock  R1Axis=[0,0,-1]
  Revolute5 : mblibv1/Joints/Revolute  LConnTagsString=__newl0|SA1  RConnTagsString=__newr0  UpdateFromCAD=on  PMImportedID=KR16L1-1:-:KR16L2-1  NumSAPorts=1  CutJoint=off  MarkAsCut=off  Primitives=prismatic  PrimitiveProps=R1$World$[0,0,1]$revolute  DialogClass=JointBlock  R1Axis=[0,0,1]
  Revolute6 : mblibv1/Joints/Revolute  LConnTagsString=__newl0  RConnTagsString=__newr0  UpdateFromCAD=on  PMImportedID=标准垫高块-1:-:轮毂工作台-2  NumSAPorts=0  CutJoint=off  MarkAsCut=off  Primitives=prismatic  PrimitiveProps=R1$WORLD$[0,1,0]$revolute  DialogClass=JointBlock  R1Axis=[0,1,0]
  Revolute7 : mblibv1/Joints/Revolute  LConnTagsString=__newl0|SA1  RConnTagsString=__newr0  UpdateFromCAD=on  PMImportedID=KR16L3-1:-:KR16L4-1  NumSAPorts=1  CutJoint=off  MarkAsCut=off  Primitives=prismatic  PrimitiveProps=R1$World$[1,6.72099e-11,0]$revolute  DialogClass=JointBlock  R1Axis=[1,6.72099e-11,0]
  Revolute8 : mblibv1/Joints/Revolute  LConnTagsString=__newl0|SA1  RConnTagsString=__newr0  UpdateFromCAD=on  PMImportedID=KR16L1-1:-:KR16底座-1  NumSAPorts=1  CutJoint=off  MarkAsCut=off  Primitives=prismatic  PrimitiveProps=R1$World$[0,1,0]$revolute  DialogClass=JointBlock  R1Axis=[0,1,0]
  RootGround : mblibv1/Bodies/Ground  UpdateFromCAD=on  PMImportedID=RootGround  LeftPortType=env  RightPortType=workingframe  PhysicalDomain=Mechanical  DialogClass=GroundBlock  CoordPosition=[0.0474298,0.716499,0.39185]  CoordPositionUnits=m  StateVectorMgrId=0  MachineId=[1 0]  ShowEnvPort=on  ParameterChecksum=[2540997710, 1269575317, 2788379925, 453987755]  TopologyChecksum=[1555649408, 2930497629, 2991550581, 636700668]
  RootPart : mblibv1/Bodies/Body  LConnTagsString=CS7|CS8|CS9|CS10  RConnTagsString=CS2|CS3|CS4|CS5|CS6  UpdateFromCAD=on  PMImportedID=KUKA-KR16-汽车轮毂/RootPart  DialogClass=MechanicalBodyBlock  Mass=0  MassUnits=kg  InertiaUnits=kg*m^2  Inertia=[0,0,0;0,0,0;0,0,0]  Shape=Cylinder  ShapeDims=[1 1]  ShapeUnits=m  ShapeUse=false  Density=1  DensityUnits=kg/m^3  DensityUse=false  GraphicsMode=MACHINE_DEFAULT  BodyColorSelMode=MACHINE_DEFAULT  BodyColor=[1;0;0]  AttachedToCS=CS1  CG=Right$CG$[0.0474298 0.716499 0.39185]$WORLD$WORLD$m$[1 0 0;0 1 0;0 0 1]$3x3 Transform$rad$WORLD$false$KUKA-KR16-汽车轮毂/RootPart::CG(AUTOGEN)  WorkingFrames=Right$CS1$[0 0 0]$WORLD$WORLD$m$[1 0 0;0 1 0;0 0 1]$3x3 Transform$rad$WORLD$false$KUKA-KR16-汽车轮毂/RootPart::CS1(AUTOGEN)#Right$CS2$[-0.021885 0.382836 1.2848]$WORLD$WORLD$m$[1 0 0;0 1 0;0 0 1]$3x3 Transform$rad$WORLD$true$KUKA-KR16-汽车轮毂/RootPart:-:轮毂工作台-2::KUKA-KR16-汽车轮毂/RootPart(AUTOGEN)#Right$CS3$[-0.0218647 1.00738 1.28478]$WORLD$WORLD$m$[1 0 0;0 1 0;0 0 1]$3x3 Transform$rad$WORLD$true$KUKA-KR16-汽车轮毂/RootPart:-:轮毂-1::KUKA-KR16-汽车轮毂/RootPart(AUTOGEN)#Right$CS4$[0 0.224865 -6.57896e-09]$WORLD$WORLD$m$[1 0 0;0 1 0;0 0 1]$3x3 Transform$rad$WORLD$true$KUKA-KR16-汽车轮毂/RootPart:-:机器人底座-1::KUKA-KR16-汽车轮毂/RootPart(AUTOGEN)#Right$CS5$[-0.021885 0.865672 1.2848]$WORLD$WORLD$m$[1 0 0;0 1 0;0 0 1]$3x3 Transform$rad$WORLD$true$KUKA-KR16-汽车轮毂/RootPart:-:标准垫高块-1::KUKA-KR16-汽车轮毂/RootPart(AUTOGEN)#Right$CS6$[0 0 0]$WORLD$WORLD$m$[1 0 0;0 1 0;0 0 1]$3x3 Transform$rad$WORLD$true$:-:KUKA-KR16-汽车轮毂/RootPart::KUKA-KR16-汽车轮毂/RootPart(AUTOGEN)#Left$CS7$[-0.021885 0 1.2848]$WORLD$WORLD$m$[1 0 0;0 1 0;0 0 1]$3x3 Transform$rad$WORLD$true$:-:KUKA-KR16-汽车轮毂/RootPart::KUKA-KR16-汽车轮毂/RootPart(AUTOGEN)#Left$CS8$[0 0.48 0]$WORLD$WORLD$m$[1 0 0;0 1 0;0 0 1]$3x3 Transform$rad$WORLD$true$:-:KUKA-KR16-汽车轮毂/RootPart::KUKA-KR16-汽车轮毂/RootPart(AUTOGEN)#Left$CS9$[0 0.5 0]$WORLD$WORLD$m$[1 0 0;0 1 0;0 0 1]$3x3 Transform$rad$WORLD$true$:-:KUKA-KR16-汽车轮毂/RootPart::KUKA-KR16-汽车轮毂/RootPart(AUTOGEN)#Left$CS10$[0.0474298 0.716499 0.39185]$WORLD$WORLD$m$[1 0 0;0 1 0;0 0 1]$3x3 Transform$rad$WORLD$true$KUKA-KR16-汽车轮毂/RootPart:-:RootGround::KUKA-KR16-汽车轮毂/RootPart(AUTOGEN)  CGPos=[0.0474298 0.716499 0.39185]  CGRot=[1 0 0;0 1 0;0 0 1]  CS0Pos=[]  CS0Rot=[]  CS1Pos=[0 0 0]  CS1Rot=[1 0 0;0 1 0;0 0 1]  CS2Pos=[-0.021885 0.382836 1.2848]  CS2Rot=[1 0 0;0 1 0;0 0 1]  CS3Pos=[-0.0218647 1.00738 1.28478]  CS3Rot=[1 0 0;0 1 0;0 0 1]  CS4Pos=[0 0.224865 -6.57896e-09]  CS4Rot=[1 0 0;0 1 0;0 0 1]  CS5Pos=[-0.021885 0.865672 1.2848]  CS5Rot=[1 0 0;0 1 0;0 0 1]  CS6Pos=[0 0 0]  CS6Rot=[1 0 0;0 1 0;0 0 1]  CS7Pos=[-0.021885 0 1.2848]  CS7Rot=[1 0 0;0 1 0;0 0 1]  CS8Pos=[0 0.48 0]  CS8Rot=[1 0 0;0 1 0;0 0 1]  CS9Pos=[0 0.5 0]  CS9Rot=[1 0 0;0 1 0;0 0 1]  CS10Pos=[0.0474298 0.716499 0.39185]  CS10Rot=[1 0 0;0 1 0;0 0 1]  CS11Pos=[]  CS11Rot=[]  CS12Pos=[]  CS12Rot=[]  CS13Pos=[]  CS13Rot=[]  CS14Pos=[]  CS14Rot=[]  CS15Pos=[]  CS15Rot=[]  CS16Pos=[]  CS16Rot=[]  CS17Pos=[]  CS17Rot=[]  CS18Pos=[]  CS18Rot=[]  CS19Pos=[]  CS19Rot=[]  CS20Pos=[]  CS20Rot=[]
  Weld : mblibv1/Joints/Weld  LConnTagsString=__newl0  RConnTagsString=__newr0  UpdateFromCAD=on  PMImportedID=KUKA-KR16-汽车轮毂/RootPart:-:轮毂工作台-2  NumSAPorts=0  CutJoint=off  MarkAsCut=off  Primitives=weld  PrimitiveProps=W$WORLD$[0.57735,0.57735,0.57735]$weld  DialogClass=JointBlock  WAxis=[0.57735,0.57735,0.57735]
  Weld1 : mblibv1/Joints/Weld  LConnTagsString=__newl0  RConnTagsString=__newr0  UpdateFromCAD=on  PMImportedID=KUKA-KR16-汽车轮毂/RootPart:-:轮毂-1  NumSAPorts=0  CutJoint=off  MarkAsCut=off  Primitives=weld  PrimitiveProps=W$WORLD$[0.57735,0.57735,0.57735]$weld  DialogClass=JointBlock  WAxis=[0.57735,0.57735,0.57735]
  Weld2 : mblibv1/Joints/Weld  LConnTagsString=__newl0  RConnTagsString=__newr0  UpdateFromCAD=on  PMImportedID=KUKA-KR16-汽车轮毂/RootPart:-:机器人底座-1  NumSAPorts=0  CutJoint=off  MarkAsCut=off  Primitives=weld  PrimitiveProps=W$WORLD$[0.57735,0.57735,0.57735]$weld  DialogClass=JointBlock  WAxis=[0.57735,0.57735,0.57735]
  Weld3 : mblibv1/Joints/Weld  LConnTagsString=__newl0  RConnTagsString=__newr0  UpdateFromCAD=on  PMImportedID=KUKA-KR16-汽车轮毂/RootPart:-:标准垫高块-1  NumSAPorts=0  CutJoint=off  MarkAsCut=off  Primitives=weld  PrimitiveProps=W$WORLD$[0.57735,0.57735,0.57735]$weld  DialogClass=JointBlock  WAxis=[0.57735,0.57735,0.57735]
  Weld4 : mblibv1/Joints/Weld  LConnTagsString=__newl0  RConnTagsString=__newr0  UpdateFromCAD=on  PMImportedID=:-:KUKA-KR16-汽车轮毂/RootPart  NumSAPorts=0  CutJoint=off  MarkAsCut=off  Primitives=weld  PrimitiveProps=W$WORLD$[0.57735,0.57735,0.57735]$weld  DialogClass=JointBlock  WAxis=[0.57735,0.57735,0.57735]
  Weld5 : mblibv1/Joints/Weld  LConnTagsString=__newl0  RConnTagsString=__newr0  UpdateFromCAD=on  PMImportedID=:-:KUKA-KR16-汽车轮毂/RootPart  NumSAPorts=0  CutJoint=off  MarkAsCut=off  Primitives=weld  PrimitiveProps=W$WORLD$[0.57735,0.57735,0.57735]$weld  DialogClass=JointBlock  WAxis=[0.57735,0.57735,0.57735]
  Weld6 : mblibv1/Joints/Weld  LConnTagsString=__newl0  RConnTagsString=__newr0  UpdateFromCAD=on  PMImportedID=KUKA-KR16-汽车轮毂/RootPart:-:RootGround  NumSAPorts=0  CutJoint=off  MarkAsCut=off  Primitives=weld  PrimitiveProps=W$WORLD$[0.57735,0.57735,0.57735]$weld  DialogClass=JointBlock  WAxis=[0.57735,0.57735,0.57735]
  机器人底座-1 : mblibv1/Bodies/Body  LConnTagsString=CS2  RConnTagsString=CS3|CS4  UpdateFromCAD=on  PMImportedID=机器人底座-1  DialogClass=MechanicalBodyBlock  Mass=49.3665  MassUnits=kg  InertiaUnits=kg*m^2  Inertia=[2.17186,0,0;0,1.46237,-7.00106e-08;0,-7.00106e-08,2.17186]  Shape=Cylinder  ShapeDims=[1 1]  ShapeUnits=m  ShapeUse=false  Density=1  DensityUnits=kg/m^3  DensityUse=false  GraphicsMode=GFXFILE  GraphicsFileName=KUKA-KR16-汽车轮毂 - 机器人底座-1.STL  BodyColorSelMode=COLORPALETTE  BodyColor=[0.501961;0.501961;0.501961]  AttachedToCS=CS1  CG=Right$CG$[0 0.224865 -6.57896e-09]$WORLD$WORLD$m$[-1 0 0;0 1 0;0 0 -1]$3x3 Transform$rad$WORLD$false$机器人底座-1::CG(AUTOGEN)  WorkingFrames=Right$CS1$[0 0.48 0]$WORLD$WORLD$m$[-1 0 0;0 1 0;0 0 -1]$3x3 Transform$rad$WORLD$false$机器人底座-1::CS1(AUTOGEN)#Left$CS2$[0 0.224865 -6.57896e-09]$WORLD$WORLD$m$[1 0 0;0 1 0;0 0 1]$3x3 Transform$rad$WORLD$true$KUKA-KR16-汽车轮毂/RootPart:-:机器人底座-1::机器人底座-1(AUTOGEN)#Right$CS3$[0 0.48 0]$WORLD$WORLD$m$[1 0 0;0 1 0;0 0 1]$3x3 Transform$rad$WORLD$true$:-:KUKA-KR16-汽车轮毂/RootPart::机器人底座-1(AUTOGEN)#Right$CS4$[0 0.5 0]$WORLD$WORLD$m$[1 0 0;0 1 0;0 0 1]$3x3 Transform$rad$WORLD$true$KR16底座-1:-:机器人底座-1::机器人底座-1(AUTOGEN)  CGPos=[0 0.224865 -6.57896e-09]  CGRot=[-1 0 0;0 1 0;0 0 -1]  CS0Pos=[]  CS0Rot=[]  CS1Pos=[0 0.48 0]  CS1Rot=[-1 0 0;0 1 0;0 0 -1]  CS2Pos=[0 0.224865 -6.57896e-09]  CS2Rot=[1 0 0;0 1 0;0 0 1]  CS3Pos=[0 0.48 0]  CS3Rot=[1 0 0;0 1 0;0 0 1]  CS4Pos=[0 0.5 0]  CS4Rot=[1 0 0;0 1 0;0 0 1]  CS5Pos=[]  CS5Rot=[]  CS6Pos=[]  CS6Rot=[]  CS7Pos=[]  CS7Rot=[]  CS8Pos=[]  CS8Rot=[]  CS9Pos=[]  CS9Rot=[]  CS10Pos=[]  CS10Rot=[]  CS11Pos=[]  CS11Rot=[]  CS12Pos=[]  CS12Rot=[]  CS13Pos=[]  CS13Rot=[]  CS14Pos=[]  CS14Rot=[]  CS15Pos=[]  CS15Rot=[]  CS16Pos=[]  CS16Rot=[]  CS17Pos=[]  CS17Rot=[]  CS18Pos=[]  CS18Rot=[]  CS19Pos=[]  CS19Rot=[]  CS20Pos=[]  CS20Rot=[]
  标准垫高块-1 : mblibv1/Bodies/Body  LConnTagsString=CS2|CS4  RConnTagsString=CS3  UpdateFromCAD=on  PMImportedID=标准垫高块-1  DialogClass=MechanicalBodyBlock  Mass=2.16  MassUnits=kg  InertiaUnits=kg*m^2  Inertia=[0.065448,0,0;0,0.116496,0;0,0,0.065448]  Shape=Cylinder  ShapeDims=[1 1]  ShapeUnits=m  ShapeUse=false  Density=1  DensityUnits=kg/m^3  DensityUse=false  GraphicsMode=GFXFILE  GraphicsFileName=KUKA-KR16-汽车轮毂 - 标准垫高块-1.STL  BodyColorSelMode=COLORPALETTE  BodyColor=[0.901961;0.901961;0.901961]  AttachedToCS=CS1  CG=Right$CG$[-0.021885 0.865672 1.2848]$WORLD$WORLD$m$[0.913076 0 -0.40779;0 1 0;0.40779 0 0.913076]$3x3 Transform$rad$WORLD$false$标准垫高块-1::CG(AUTOGEN)  WorkingFrames=Right$CS1$[-0.021885 0.765672 1.2848]$WORLD$WORLD$m$[0.913076 0 -0.40779;0 1 0;0.40779 0 0.913076]$3x3 Transform$rad$WORLD$false$标准垫高块-1::CS1(AUTOGEN)#Left$CS2$[-0.021885 0.865672 1.2848]$WORLD$WORLD$m$[1 0 0;0 1 0;0 0 1]$3x3 Transform$rad$WORLD$true$KUKA-KR16-汽车轮毂/RootPart:-:标准垫高块-1::标准垫高块-1(AUTOGEN)#Right$CS3$[-0.021885 0.965672 1.2848]$WORLD$WORLD$m$[1 0 0;0 1 0;0 0 1]$3x3 Transform$rad$WORLD$true$标准垫高块-1:-:轮毂-1::标准垫高块-1(AUTOGEN)#Left$CS4$[-0.021885 0.765672 1.2848]$WORLD$WORLD$m$[1 0 0;0 1 0;0 0 1]$3x3 Transform$rad$WORLD$true$标准垫高块-1:-:轮毂工作台-2::标准垫高块-1(AUTOGEN)  CGPos=[-0.021885 0.865672 1.2848]  CGRot=[0.913076 0 -0.40779;0 1 0;0.40779 0 0.913076]  CS0Pos=[]  CS0Rot=[]  CS1Pos=[-0.021885 0.765672 1.2848]  CS1Rot=[0.913076 0 -0.40779;0 1 0;0.40779 0 0.913076]  CS2Pos=[-0.021885 0.865672 1.2848]  CS2Rot=[1 0 0;0 1 0;0 0 1]  CS3Pos=[-0.021885 0.965672 1.2848]  CS3Rot=[1 0 0;0 1 0;0 0 1]  CS4Pos=[-0.021885 0.765672 1.2848]  CS4Rot=[1 0 0;0 1 0;0 0 1]  CS5Pos=[]  CS5Rot=[]  CS6Pos=[]  CS6Rot=[]  CS7Pos=[]  CS7Rot=[]  CS8Pos=[]  CS8Rot=[]  CS9Pos=[]  CS9Rot=[]  CS10Pos=[]  CS10Rot=[]  CS11Pos=[]  CS11Rot=[]  CS12Pos=[]  CS12Rot=[]  CS13Pos=[]  CS13Rot=[]  CS14Pos=[]  CS14Rot=[]  CS15Pos=[]  CS15Rot=[]  CS16Pos=[]  CS16Rot=[]  CS17Pos=[]  CS17Rot=[]  CS18Pos=[]  CS18Rot=[]  CS19Pos=[]  CS19Rot=[]  CS20Pos=[]  CS20Rot=[]
  轮毂-1 : mblibv1/Bodies/Body  LConnTagsString=CS2|CS3|CS4  UpdateFromCAD=on  PMImportedID=轮毂-1  DialogClass=MechanicalBodyBlock  Mass=9.03222  MassUnits=kg  InertiaUnits=kg*m^2  Inertia=[0.170691,-4.48638e-05,-6.58631e-06;-4.48638e-05,0.171308,-1.12365e-05;-6.58631e-06,-1.12365e-05,0.334242]  Shape=Cylinder  ShapeDims=[1 1]  ShapeUnits=m  ShapeUse=false  Density=1  DensityUnits=kg/m^3  DensityUse=false  GraphicsMode=GFXFILE  GraphicsFileName=KUKA-KR16-汽车轮毂 - 轮毂-1.STL  BodyColorSelMode=COLORPALETTE  BodyColor=[0.8;0.8;0.8]  AttachedToCS=CS1  CG=Right$CG$[-0.0218647 1.00738 1.28478]$WORLD$WORLD$m$[-0.997001 -0.0773949 0;0 0 1;-0.0773949 0.997001 0]$3x3 Transform$rad$WORLD$false$轮毂-1::CG(AUTOGEN)  WorkingFrames=Right$CS1$[-0.021885 0.965672 1.2848]$WORLD$WORLD$m$[-0.997001 -0.0773949 0;0 0 1;-0.0773949 0.997001 0]$3x3 Transform$rad$WORLD$false$轮毂-1::CS1(AUTOGEN)#Left$CS2$[-0.0218647 1.00738 1.28478]$WORLD$WORLD$m$[1 0 0;0 1 0;0 0 1]$3x3 Transform$rad$WORLD$true$KUKA-KR16-汽车轮毂/RootPart:-:轮毂-1::轮毂-1(AUTOGEN)#Left$CS3$[0 0 0]$WORLD$WORLD$m$[1 0 0;0 1 0;0 0 1]$3x3 Transform$rad$WORLD$true$:-:KUKA-KR16-汽车轮毂/RootPart::轮毂-1(AUTOGEN)#Left$CS4$[-0.021885 0.965672 1.2848]$WORLD$WORLD$m$[1 0 0;0 1 0;0 0 1]$3x3 Transform$rad$WORLD$true$标准垫高块-1:-:轮毂-1::轮毂-1(AUTOGEN)  CGPos=[-0.0218647 1.00738 1.28478]  CGRot=[-0.997001 -0.0773949 0;0 0 1;-0.0773949 0.997001 0]  CS0Pos=[]  CS0Rot=[]  CS1Pos=[-0.021885 0.965672 1.2848]  CS1Rot=[-0.997001 -0.0773949 0;0 0 1;-0.0773949 0.997001 0]  CS2Pos=[-0.0218647 1.00738 1.28478]  CS2Rot=[1 0 0;0 1 0;0 0 1]  CS3Pos=[0 0 0]  CS3Rot=[1 0 0;0 1 0;0 0 1]  CS4Pos=[-0.021885 0.965672 1.2848]  CS4Rot=[1 0 0;0 1 0;0 0 1]  CS5Pos=[]  CS5Rot=[]  CS6Pos=[]  CS6Rot=[]  CS7Pos=[]  CS7Rot=[]  CS8Pos=[]  CS8Rot=[]  CS9Pos=[]  CS9Rot=[]  CS10Pos=[]  CS10Rot=[]  CS11Pos=[]  CS11Rot=[]  CS12Pos=[]  CS12Rot=[]  CS13Pos=[]  CS13Rot=[]  CS14Pos=[]  CS14Rot=[]  CS15Pos=[]  CS15Rot=[]  CS16Pos=[]  CS16Rot=[]  CS17Pos=[]  CS17Rot=[]  CS18Pos=[]  CS18Rot=[]  CS19Pos=[]  CS19Rot=[]  CS20Pos=[]  CS20Rot=[]
  轮毂工作台-2 : mblibv1/Bodies/Body  LConnTagsString=CS2  RConnTagsString=CS3|CS4  UpdateFromCAD=on  PMImportedID=轮毂工作台-2  DialogClass=MechanicalBodyBlock  Mass=66.8102  MassUnits=kg  InertiaUnits=kg*m^2  Inertia=[9.55359,0,0;0,6.17657,0;0,0,9.55359]  Shape=Cylinder  ShapeDims=[1 1]  ShapeUnits=m  ShapeUse=false  Density=1  DensityUnits=kg/m^3  DensityUse=false  GraphicsMode=GFXFILE  GraphicsFileName=KUKA-KR16-汽车轮毂 - 轮毂工作台-2.STL  BodyColorSelMode=COLORPALETTE  BodyColor=[0.50196 0.50196 0.50196]  AttachedToCS=CS1  CG=Right$CG$[-0.021885 0.382836 1.2848]$WORLD$WORLD$m$[1 0 0;0 1 0;0 0 1]$3x3 Transform$rad$WORLD$false$轮毂工作台-2::CG(AUTOGEN)  WorkingFrames=Right$CS1$[-0.021885 0 1.2848]$WORLD$WORLD$m$[1 0 0;0 1 0;0 0 1]$3x3 Transform$rad$WORLD$false$轮毂工作台-2::CS1(AUTOGEN)#Left$CS2$[-0.021885 0.382836 1.2848]$WORLD$WORLD$m$[1 0 0;0 1 0;0 0 1]$3x3 Transform$rad$WORLD$true$KUKA-KR16-汽车轮毂/RootPart:-:轮毂工作台-2::轮毂工作台-2(AUTOGEN)#Right$CS3$[-0.021885 0 1.2848]$WORLD$WORLD$m$[1 0 0;0 1 0;0 0 1]$3x3 Transform$rad$WORLD$true$:-:KUKA-KR16-汽车轮毂/RootPart::轮毂工作台-2(AUTOGEN)#Right$CS4$[-0.021885 0.765672 1.2848]$WORLD$WORLD$m$[1 0 0;0 1 0;0 0 1]$3x3 Transform$rad$WORLD$true$标准垫高块-1:-:轮毂工作台-2::轮毂工作台-2(AUTOGEN)  CGPos=[-0.021885 0.382836 1.2848]  CGRot=[1 0 0;0 1 0;0 0 1]  CS0Pos=[]  CS0Rot=[]  CS1Pos=[-0.021885 0 1.2848]  CS1Rot=[1 0 0;0 1 0;0 0 1]  CS2Pos=[-0.021885 0.382836 1.2848]  CS2Rot=[1 0 0;0 1 0;0 0 1]  CS3Pos=[-0.021885 0 1.2848]  CS3Rot=[1 0 0;0 1 0;0 0 1]  CS4Pos=[-0.021885 0.765672 1.2848]  CS4Rot=[1 0 0;0 1 0;0 0 1]  CS5Pos=[]  CS5Rot=[]  CS6Pos=[]  CS6Rot=[]  CS7Pos=[]  CS7Rot=[]  CS8Pos=[]  CS8Rot=[]  CS9Pos=[]  CS9Rot=[]  CS10Pos=[]  CS10Rot=[]  CS11Pos=[]  CS11Rot=[]  CS12Pos=[]  CS12Rot=[]  CS13Pos=[]  CS13Rot=[]  CS14Pos=[]  CS14Rot=[]  CS15Pos=[]  CS15Rot=[]  CS16Pos=[]  CS16Rot=[]  CS17Pos=[]  CS17Rot=[]  CS18Pos=[]  CS18Rot=[]  CS19Pos=[]  CS19Rot=[]  CS20Pos=[]  CS20Rot=[]
  Conn1 : PMIOPort  Port=1  Side=Right
  wires:
  Add1/1 -> Mux2/1
  Demux1/1 -> Mux/2
  Demux1/7 -> Mux6/2
  Mux2/1 -> Joint Actuator2/1
  Demux/3 -> Add1/2
  Constant1/1 -> Add1/1
  Demux2/2 -> Mux1/3
  Demux2/5 -> Mux4/3
  Add/1 -> Mux1/1
  Mux1/1 -> Joint Actuator1/1
  Demux2/3 -> Mux2/3
  Mux/1 -> Joint Actuator/1
  Gain1/1 -> Add/2
  Demux/1 -> Gain/1
  Demux2/4 -> Mux3/3
  Demux2/7 -> Mux6/3
  In3/1 -> Demux/1
  In2/1 -> Demux2/1
  In1/1 -> Demux1/1
  Demux/4 -> Mux3/1
  Mux3/1 -> Joint Actuator3/1
  Demux/2 -> Gain1/1
  Demux1/6 -> Mux5/2
  Demux1/2 -> Mux1/2
  Mux6/1 -> Joint Actuator6/1
  Demux/7 -> Mux6/1
  Constant/1 -> Add/1
  Gain2/1 -> Mux4/1
  Gain/1 -> Mux/1
  Demux/5 -> Gain2/1
  Mux4/1 -> Joint Actuator4/1
  Demux2/1 -> Mux/3
  Demux2/6 -> Mux5/3
  Demux1/3 -> Mux2/2
  Demux1/5 -> Mux4/2
  Demux/6 -> Mux5/1
  Mux5/1 -> Joint Actuator5/1
  Demux1/4 -> Mux3/2
  connections:
  Joint Actuator2/RConn1 -- Revolute4/LConn2
  Joint Actuator1/RConn1 -- Revolute5/LConn2
  Conn1/RConn1 -- KR16电主轴-1/RConn1
  Joint Actuator3/RConn1 -- Revolute7/LConn2
  Revolute/LConn2 -- Joint Actuator6/RConn1
  Joint Actuator/RConn1 -- Revolute8/LConn2
  Revolute2/LConn2 -- Joint Actuator4/RConn1
  RootPart/RConn1 -- Weld/LConn1
  KR16底座-1/RConn1 -- Planar/LConn1
  轮毂工作台-2/RConn2 -- Revolute6/LConn1
  Weld2/RConn1 -- 机器人底座-1/LConn1
  RootPart/RConn4 -- Weld3/LConn1
  RootPart/RConn5 -- Custom Joint/LConn1
  机器人底座-1/RConn1 -- Weld5/LConn1
  轮毂工作台-2/RConn1 -- Weld4/LConn1
  Revolute/RConn1 -- KR16电主轴-1/LConn1
  标准垫高块-1/RConn1 -- Revolute1/LConn1
  Weld3/RConn1 -- 标准垫高块-1/LConn1
  Revolute1/RConn1 -- 轮毂-1/LConn3
  Weld4/RConn1 -- RootPart/LConn1
  KR16L6-3/RConn1 -- Revolute/LConn1
  Weld/RConn1 -- 轮毂工作台-2/LConn1
  Weld5/RConn1 -- RootPart/LConn2
  RootPart/RConn2 -- Weld1/LConn1
  Revolute3/RConn1 -- KR16L6-3/LConn1
  RootPart/RConn3 -- Weld2/LConn1
  KR16L2-1/RConn1 -- Revolute4/LConn1
  Revolute4/RConn1 -- KR16L3-1/LConn1
  Revolute2/RConn1 -- KR16L5-1/LConn1
  KR16L4-1/RConn1 -- Revolute2/LConn1
  KR16L1-1/RConn1 -- Revolute5/LConn1
  Revolute5/RConn1 -- KR16L2-1/LConn1
  KR16L5-1/RConn1 -- Revolute3/LConn1
  Weld1/RConn1 -- 轮毂-1/LConn1
  Planar/RConn1 -- RootPart/LConn3
  Custom Joint/RConn1 -- 轮毂-1/LConn2
  机器人底座-1/RConn2 -- Prismatic/LConn1
  RootGround/RConn1 -- Weld6/LConn1
  Prismatic/RConn1 -- KR16底座-1/LConn1
  KR16L3-1/RConn1 -- Revolute7/LConn1
  Revolute8/RConn1 -- KR16L1-1/LConn1
  KR16底座-1/RConn2 -- Revolute8/LConn1
  RootGround/LConn1 -- Machine Environment/RConn1
  Revolute6/RConn1 -- 标准垫高块-1/LConn2
  Revolute7/RConn1 -- KR16L4-1/LConn1
  Weld6/RConn1 -- RootPart/LConn4
  Joint Actuator5/RConn1 -- Revolute3/LConn2
